simulink model "simexa25"  (Simulink 4.00)
settings: Solver=ode45  SolverMode=SingleTasking  StartTime=0.0  StopTime=100.0  RelTol=1e-3  AbsTol=1e-6
libraries: simulink3 x1
settings Model: LastModifiedBy=saadat  LimitDataPoints=off  RTWTemplateMakefile=grt_vc.tmf  ExtModeTrigMode=oneshot  ExtModeArmWhenConnect=off

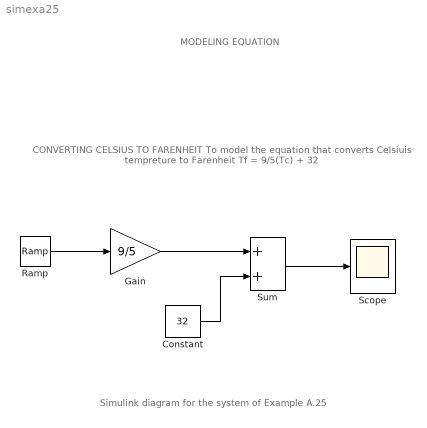
== system simexa25 ==
  note: Simulink diagram for the system of Example A.25
  note: CONVERTING CELSIUS TO FARENHEIT
      |
      | To model the equation that converts Celsiuis tempreture to Farenheit
      |
      | Tf = 9/5(Tc) + 32
  note: MODELING EQUATION
  Constant : Constant  Value=32
  Gain : Gain  Gain=9/5  Multiplication=Element-wise(K.*u)  SaturateOnIntegerOverflow=on
  Ramp : simulink3/Sources/Ramp  slope=1  start=0  X0=0
  Scope : Scope
      settings: TickLabels=on  TimeRange=auto  YMin=-5  YMax=5  SaveToWorkspace=off  SaveName=ScopeData  DataFormat=Array  LimitDataPoints=on  MaxDataPoints=5000
  Sum : Sum  Inputs=++  SaturateOnIntegerOverflow=on
  wires:
  Ramp/1 -> Gain/1
  Gain/1 -> Sum/1
  Sum/1 -> Scope/1
  Constant/1 -> Sum/2
